simulink model "haya_cvt_multiple_gear"  (R2020a)
settings: Solver=VariableStepAuto  StartTime=0.0  StopTime=10.0  RelTol=1e-3
libraries: fl_lib x19, nesl_utility x9, sdl_lib x9, simulink x2
settings Model: Creator=kishan  LastModifiedBy=kishan

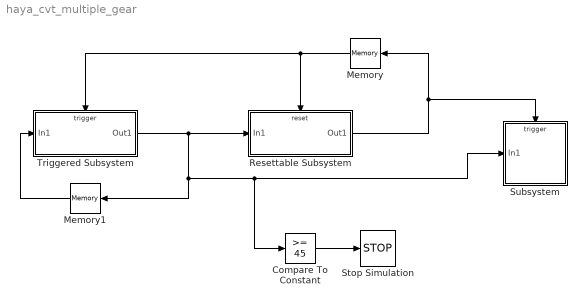
== system haya_cvt_multiple_gear ==
  Compare To Constant : simulink/Logic and Bit Operations/Compare To Constant  relop=>=  const=45  OutDataTypeStr=boolean
  Memory : Memory
  Memory1 : Memory  InitialCondition=6.9
  Resettable Subsystem : Subsystem  TreatAsAtomicUnit=on
  Stop Simulation : Stop
  Subsystem : Subsystem
  Triggered Subsystem : Subsystem  TreatAsAtomicUnit=on
  wires:
  Resettable Subsystem/1(Out1) -> Memory/1, Subsystem/Trigger
  Triggered Subsystem/1(Out1) -> Memory1/1, Compare To Constant/1, Subsystem/1(In1), Resettable Subsystem/1(In1)
  Compare To Constant/1 -> Stop Simulation/1
  Memory/1 -> Triggered Subsystem/Trigger, Resettable Subsystem/Reset
  Memory1/1 -> Triggered Subsystem/1(In1)

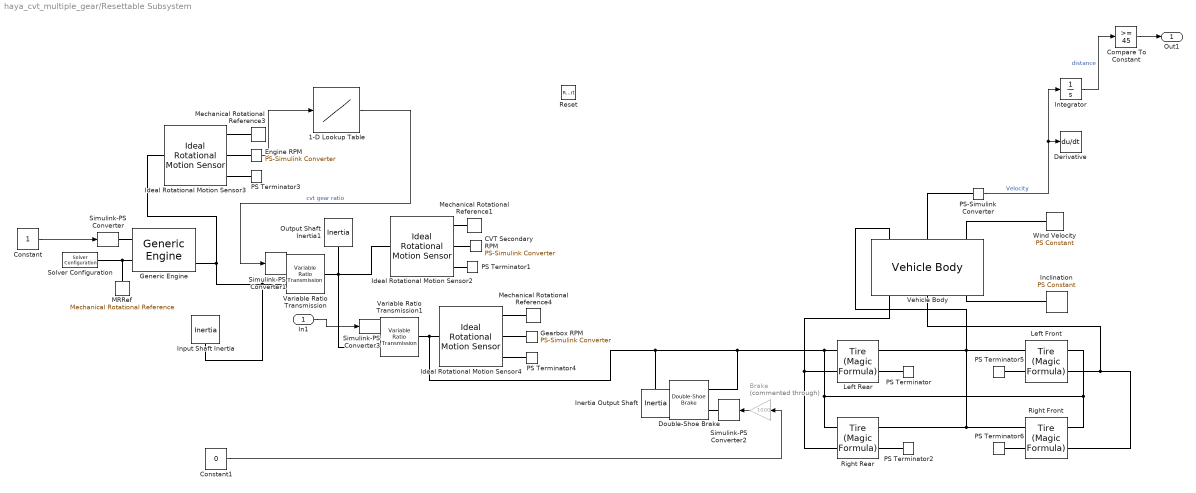
== system haya_cvt_multiple_gear/Resettable Subsystem ==
  In1 : Inport
  Reset : ResetPort  DisableCoverage=on
  1-D Lookup Table : Lookup_n-D  NumberOfTableDimensions=1  BreakpointsForDimension1=[1200, 1300, 1400, 1500, 1600, 1700, 1800, 2000, 2200, 2400, 2600, 2800, 3000, 3200, 3400, 3600, 3800]  Table=[3.9, 3.9, 3.9, 3.9, 3.9, 3.9, 3.9, 3.75, 3.5, 3.2, 2.8, 1.4, 1, 0.9, 0.9, 0.9, 0.9]  InternalRulePriority=Speed  RndMeth=Simplest  InputSameDT=on
  Brake : Gain  Commented=through  Gain=1000
  CVT Secondary RPM : nesl_utility/PS-Simulink Converter  PhysicalDomain=network_engine_domain  SubClassName=ps_output  LeftPortType=input  RightPortType=output  PseudoPeriodic=off  Frequencies=[]  Unit=rpm  AffineConversion=off
  Compare To Constant : simulink/Logic and Bit Operations/Compare To Constant  relop=>=  const=45  OutDataTypeStr=boolean
  Constant : Constant
  Constant1 : Constant  Value=0
  Derivative : Derivative
  Double-Shoe Brake : sdl_lib/Brakes & Detents/Rotational/Double-Shoe Brake  r_drum=150 mm  r_act=100 mm  r_pin=125 mm  theta_pin=15 deg  theta_0=5 deg  theta_shoe=120 deg  mu_visc=.01 N*m/(rad/s)  thermal_port=simscape.enum.thermaleffects.omit  mu=0.3  temperature_TLU=[280.0, 300.0, 320.0] K  mu_TLU=[0.1, 0.05, 0.03]  thermal_mass=50 kJ/K  w_thr=0.01 rad/s  temperature_specify=off  temperature_priority=High  temperature=300 K  temperature_nominal_specify=off  temperature_nominal_unit=K  temperature_nominal_value=1
      settings: SourceProductBaseCode=LD  InternalSimscapePortConfiguration="{\"Bottom\":[],\"Left\":[{\"id\":\"F\",\"label\":\"F\",\"type\":\"input\"},{\"id\":\"S\",\"label\":\"S\",\"type\":\"foundation.mechanical.rotational.rotational\"}],\"Right\":[],\"Top\":[]}"
  Engine RPM : nesl_utility/PS-Simulink Converter  PhysicalDomain=network_engine_domain  SubClassName=ps_output  LeftPortType=input  RightPortType=output  PseudoPeriodic=off  Frequencies=[]  Unit=rpm  AffineConversion=off
  Gearbox RPM : nesl_utility/PS-Simulink Converter  PhysicalDomain=network_engine_domain  SubClassName=ps_output  LeftPortType=input  RightPortType=output  PseudoPeriodic=off  Frequencies=[]  Unit=rpm  AffineConversion=off
  Generic Engine : sdl_lib/Engines/Generic Engine  model_parameterization=2  engine_type=1  P_max=10 HP_DIN  w_P_max=3600 rpm  w_max=3800 rpm  w_min=2000 rpm  w_tab=[1200,1300,1400,1500,1600,1700,1800,1900,1999.91475361355,2037.58825921408,2067.14428302096,2107.1635059702,2136.68404125541,2172.52153339987,2199.90684263059,2233.66234150309,2279.96303278992,2322.09973753281,2353.6667775683,2389.46878119108,2421.01807696573,2463.08380466526,2494.65084470075,2534.65232338915,2583.01726368711,2600,2620.86577206018,2654.46157258512,2711.22546301431,2765.81863886733,2828.84625337326,2893.92037262948,2959.01223614654,3011.45244168423,3074.37359062512,3126.8137961628,3181.31825071162,3235.80496099959,3283.9747144283,3348.94236811948,3390.79516468892,3438.92942959595,3480.79997042623,3535.25119219253,3583.33222431703] rpm  trq_tab=[2.9584703,4.1836314,5.4162917,5.69929300000000,7.851956,9.435718,10.573324,11.506594,12.169014084507,12.7323943661972,13.2394366197183,13.6338028169014,14.0281690140845,14.4788732394366,14.7605633802817,15.2676056338028,15.6056338028169,16.056338028169,16.2816901408451,16.6197183098592,16.7887323943662,17.0140845070423,17.2394366197183,17.5774647887324,17.8028169014085,17.9718309859155,17.9718309859155,18.1971830985916,18.1971830985916,18.5098591549296,19,18.5535211267606,18.2535211267606,18.0845070422535,17.8591549295775,17.6901408450704,17.4084507042254,17.0704225352113,16.6760563380282,16.2816901408451,15.830985915493,15.3239436619718,14.9295774647887,14.4788732394366,13.8028169014085] N*m  pwr_tab=[5.25, 5.75, 6.3, 7, 7.5, 8, 8.4, 8.6, 9] kW  interp_method=simscape.enum.interpolation.smooth  model_inertia=1  inertia=0.8 kg*m^2  initial_velocity=1500 rpm  model_time_constant=1  time_constant=1 s  T0=0  w_thr=100 rpm  idle_speed=1  idle_speed_reference=1500 rpm  tau_controller=1 s  idle_w_thr=1 rpm  redline=1  redline_speed=3550 rpm  tau_redline=1 s  redline_w_thr=1 rpm  fc_model=0  fc_per_rev=25 mg/rev  displaced_volume=400 cm^3  rev_per_cycle=2  fc_w_tab=[1000, 2000, 3000, 4000, 5000, 6000] rpm  fc_trq_tab=[0, 80, 160, 200, 240, 320, 360, 400] N*m  fc_tab=[.5, .9, 1.4, 1.6, 1.9, 2.7, 3.4, 4.4; 1, 1.7, 2.7, 3.1, 3.6, 5, 6, 7.4; 1.4, 2.7, 4, 4.8, 5.6, 7.5, 8.5, 10.5; 2, 3.6, 5.8, 6.7, 8, 10.4, 11.7, 13.3; 2.5, 4.8, 7.9, 9.4, 10.8, 14, 16.2, 18.6; 3.1, 6, 10.3, 11.9, 13.8, 18.4, 22, 26.5] g/s  bmep_tab=[0, 250, 500, 625, 750, 1000, 1150, 1250] kPa  bsfc_tab=[410, 380, 300, 280, 270, 290, 320, 380; 410, 370, 290, 270, 260, 270, 285, 320; 415, 380, 290, 275, 265, 270, 270, 300; 420, 390, 310, 290, 285, 280, 280, 285; 430, 410, 340, 320, 310, 300, 310, 320; 450, 430, 370, 340, 330, 330, 350, 380] g/hr/kW  fc_interp_method=simscape.enum.interpolation.linear
      settings: SourceProductBaseCode=LD  LogSimulationData=on  InternalSimscapePortConfiguration="{\"Bottom\":[],\"Left\":[{\"id\":\"T\",\"label\":\"T\",\"type\":\"input\"},{\"id\":\"B\",\"label\":\"B\",\"type\":\"foundation.mechanical.rotational.rotational\"}],\"Right\":[{\"id\":\"P\",\"label\":\"P\",\"type\":\"output\"},{\"id\":\"FC\",\"label\":\"FC\",\"type\":\"output\"},{\"id\":\"F\",\"label\":\"F\",\"type\":\"foundation.mechanical.rotational.rotational\"}],\"Top\":[]}"
  Ideal Rotational Motion Sensor2 : fl_lib/Mechanical/Mechanical Sensors/Ideal Rotational Motion Sensor  wrap_angle=simscape.enum.onoff.off  offset=0 rad
  Ideal Rotational Motion Sensor3 : fl_lib/Mechanical/Mechanical Sensors/Ideal Rotational Motion Sensor  wrap_angle=simscape.enum.onoff.off  offset=0 rad
  Ideal Rotational Motion Sensor4 : fl_lib/Mechanical/Mechanical Sensors/Ideal Rotational Motion Sensor  wrap_angle=simscape.enum.onoff.off  offset=0 rad
  Inclination : fl_lib/Physical Signals/Sources/PS Constant  constant=0
  Inertia Output Shaft : fl_lib/Mechanical/Rotational Elements/Inertia  inertia=1e-1 kg*m^2  w_specify=on  w_priority=High  w=0 rpm  w_nominal_specify=off  w_nominal_unit=rad/s  w_nominal_value=1  t_specify=off  t_priority=High  t=0 N*m  t_nominal_specify=off  t_nominal_unit=N*m  t_nominal_value=1
  Input Shaft Inertia : fl_lib/Mechanical/Rotational Elements/Inertia  inertia=0.00253 kg*m^2  w_specify=on  w_priority=None  w=2500 rpm  w_nominal_specify=off  w_nominal_unit=rad/s  w_nominal_value=1  t_specify=off  t_priority=High  t=0 N*m  t_nominal_specify=off  t_nominal_unit=N*m  t_nominal_value=1
  Integrator : Integrator
  Left Front : sdl_lib/Tires & Vehicles/Tire (Magic Formula)  parameterization=sdl.enum.magic_tire_model.constant  F_z1=3000 N  F_x1=3500 N  kappa1=10  B_m=5  C_m=2  D_m=0.3  E_m=1  fz0=4000 N  p_Cx=1.685  p_Dx=[1.21, -.037]  p_Ex=[.344, .095, -.02, 0]  p_Kx=[21.51, -.163, .245]  p_Hx=[-.002, .002]  p_Vx=[0, 0]  v_tr_thr=0.1 m/s  r_e=0.292 m  model_compliance=0  stiffness=1e6 N/m  damping=1000 N/(m/s)  model_inertia=1  inertia=0.0667255 kg*m^2  initial_velocity=0 rpm  model_resistance=1  resistance_model=1  coeff=0.02  p_tire=250e3 Pa  alpha=-0.003  beta=0.97  coeff_a=84e-4  coeff_b=6.2e-4 s/m  coeff_c=1.6e-4 s^2/m^2  v_thr=0.001 m/s
  Left Rear : sdl_lib/Tires & Vehicles/Tire (Magic Formula)  parameterization=sdl.enum.magic_tire_model.constant  F_z1=3000 N  F_x1=3500 N  kappa1=10  B_m=5  C_m=2  D_m=0.3  E_m=1  fz0=4000 N  p_Cx=1.685  p_Dx=[1.21, -.037]  p_Ex=[.344, .095, -.02, 0]  p_Kx=[21.51, -.163, .245]  p_Hx=[-.002, .002]  p_Vx=[0, 0]  v_tr_thr=0.1 m/s  r_e=0.292 m  model_compliance=0  stiffness=1e6 N/m  damping=1000 N/(m/s)  model_inertia=1  inertia=0.0667255 kg*m^2  initial_velocity=0 rpm  model_resistance=1  resistance_model=1  coeff=0.02  p_tire=250e3 Pa  alpha=-0.003  beta=0.97  coeff_a=84e-4  coeff_b=6.2e-4 s/m  coeff_c=1.6e-4 s^2/m^2  v_thr=0.001 m/s
  MRRef : fl_lib/Mechanical/Rotational Elements/Mechanical Rotational Reference
  Mechanical Rotational Reference1 : fl_lib/Mechanical/Rotational Elements/Mechanical Rotational Reference
  Mechanical Rotational Reference3 : fl_lib/Mechanical/Rotational Elements/Mechanical Rotational Reference
  Mechanical Rotational Reference4 : fl_lib/Mechanical/Rotational Elements/Mechanical Rotational Reference
  Output Shaft Inertia1 : fl_lib/Mechanical/Rotational Elements/Inertia  inertia=0.00243 kg*m^2  w_specify=on  w_priority=None  w=2500 rpm  w_nominal_specify=off  w_nominal_unit=rad/s  w_nominal_value=1  t_specify=off  t_priority=High  t=0 N*m  t_nominal_specify=off  t_nominal_unit=N*m  t_nominal_value=1
  PS Terminator{,1..6} (7 alike) : fl_lib/Physical Signals/Sinks/PS Terminator
  PS-Simulink Converter : nesl_utility/PS-Simulink Converter  PhysicalDomain=network_engine_domain  SubClassName=ps_output  LeftPortType=input  RightPortType=output  PseudoPeriodic=off  Frequencies=[]  Unit=km/hr  AffineConversion=off
  Right Front : sdl_lib/Tires & Vehicles/Tire (Magic Formula)  parameterization=sdl.enum.magic_tire_model.constant  F_z1=3000 N  F_x1=3500 N  kappa1=10  B_m=5  C_m=2  D_m=0.3  E_m=1  fz0=4000 N  p_Cx=1.685  p_Dx=[1.21, -.037]  p_Ex=[.344, .095, -.02, 0]  p_Kx=[21.51, -.163, .245]  p_Hx=[-.002, .002]  p_Vx=[0, 0]  v_tr_thr=0.1 m/s  r_e=0.292 m  model_compliance=0  stiffness=1e6 N/m  damping=1000 N/(m/s)  model_inertia=1  inertia=0.0667255 kg*m^2  initial_velocity=0 rpm  model_resistance=1  resistance_model=1  coeff=0.02  p_tire=250e3 Pa  alpha=-0.003  beta=0.97  coeff_a=84e-4  coeff_b=6.2e-4 s/m  coeff_c=1.6e-4 s^2/m^2  v_thr=0.001 m/s
  Right Rear : sdl_lib/Tires & Vehicles/Tire (Magic Formula)  parameterization=sdl.enum.magic_tire_model.constant  F_z1=3000 N  F_x1=3500 N  kappa1=10  B_m=5  C_m=2  D_m=0.3  E_m=1  fz0=4000 N  p_Cx=1.685  p_Dx=[1.21, -.037]  p_Ex=[.344, .095, -.02, 0]  p_Kx=[21.51, -.163, .245]  p_Hx=[-.002, .002]  p_Vx=[0, 0]  v_tr_thr=0.1 m/s  r_e=0.292 m  model_compliance=0  stiffness=1e6 N/m  damping=1000 N/(m/s)  model_inertia=1  inertia=0.0667255 kg*m^2  initial_velocity=0 rpm  model_resistance=1  resistance_model=1  coeff=0.02  p_tire=250e3 Pa  alpha=-0.003  beta=0.97  coeff_a=84e-4  coeff_b=6.2e-4 s/m  coeff_c=1.6e-4 s^2/m^2  v_thr=0.001 m/s
  Simulink-PS Converter : nesl_utility/Simulink-PS Converter  PhysicalDomain=network_engine_domain  SubClassName=ps_input  LeftPortType=input  RightPortType=output  PseudoPeriodic=off  Frequencies=[]  NoiseDistribution=none  NoiseParameters=[]  Unit=1  AffineConversion=off  FilteringAndDerivatives=zero  SimscapeFilterOrder=1  InputFilterTimeConstant=0.001  UdotUserProvided=1
  Simulink-PS Converter1 : nesl_utility/Simulink-PS Converter  PhysicalDomain=network_engine_domain  SubClassName=ps_input  LeftPortType=input  RightPortType=output  PseudoPeriodic=off  Frequencies=[]  NoiseDistribution=none  NoiseParameters=[]  Unit=1  AffineConversion=off  FilteringAndDerivatives=zero  SimscapeFilterOrder=1  InputFilterTimeConstant=.001  UdotUserProvided=0
  Simulink-PS Converter2 : nesl_utility/Simulink-PS Converter  PhysicalDomain=network_engine_domain  SubClassName=ps_input  LeftPortType=input  RightPortType=output  PseudoPeriodic=off  Frequencies=[]  NoiseDistribution=none  NoiseParameters=[]  Unit=N  AffineConversion=off  FilteringAndDerivatives=zero  SimscapeFilterOrder=1  InputFilterTimeConstant=0.001  UdotUserProvided=1
  Simulink-PS Converter3 : nesl_utility/Simulink-PS Converter  PhysicalDomain=network_engine_domain  SubClassName=ps_input  LeftPortType=input  RightPortType=output  PseudoPeriodic=off  Frequencies=[]  NoiseDistribution=none  NoiseParameters=[]  Unit=1  AffineConversion=off  FilteringAndDerivatives=zero  SimscapeFilterOrder=1  InputFilterTimeConstant=0.001  UdotUserProvided=1
  Solver Configuration : nesl_utility/Solver Configuration  PhysicalDomain=network_engine_domain  SubClassName=solver  LeftPortType=input  RightPortType=generic  Tones=[]  Harmonics=[]  SimulateNoise=off  Profile=off  UseLocalSampling=off  EnableSwitchedLinearOptims=on  FrequencyDomain=off  UseCCode=off  RelTol=0.001  AbsTol=1e-06  MinStep=1e-09  ToWorkspace=off  RevertToSquareIcSolve=off  NumHomotopyIterations=100  PhasorMode=off  PhasorModeNumHarmonics=1  DoDC=off  ResidualTolerance=1e-9  UseLocalSolver=off  LocalSolverChoice=NE_BACKWARD_EULER_ADVANCER  LocalSolverSampleTime=0.001  DoFixedCost=off  MaxNonlinIter=3  MaxModeIter=2  LinearAlgebra=Sparse  EquationFormulation=NE_TIME_EF  DelaysMemoryBudget=1024  AutomaticFiltering=on  FilteringTimeConstant=0.001  PartitionStorageMethod=AS_NEEDED  PartitionMemoryBudget=1024  PartitionMethod=FAST
  Variable Ratio Transmission : sdl_lib/Couplings & Drives/Variable Ratio Transmission  rotation_direction=1  kp=3e5 N*m/rad  kv=0.05 N*m/(rad/s)  initial_torque=0 N*m  losses_model=2  efficiency=0.8  mu_visc=[0, 0] N*m/(rad/s)  w_thr=0.01 rad/s  R_specify=off  R_priority=None  R=1  R_nominal_specify=off  R_nominal_unit=1  R_nominal_value=1
      settings: SourceProductBaseCode=LD  InternalSimscapePortConfiguration="{\"Bottom\":[],\"Left\":[{\"id\":\"ratio\",\"label\":\"r\",\"type\":\"input\"},{\"id\":\"B\",\"label\":\"B\",\"type\":\"foundation.mechanical.rotational.rotational\"}],\"Right\":[{\"id\":\"F\",\"label\":\"F\",\"type\":\"foundation.mechanical.rotational.rotational\"}],\"Top\":[]}"
  Variable Ratio Transmission1 : sdl_lib/Couplings & Drives/Variable Ratio Transmission  rotation_direction=1  kp=3e5 N*m/rad  kv=0.05 N*m/(rad/s)  initial_torque=0 N*m  losses_model=2  efficiency=0.8  mu_visc=[0, 0] N*m/(rad/s)  w_thr=0.01 rad/s  R_specify=off  R_priority=None  R=1  R_nominal_specify=off  R_nominal_unit=1  R_nominal_value=1
      settings: SourceProductBaseCode=LD  InternalSimscapePortConfiguration="{\"Bottom\":[],\"Left\":[{\"id\":\"ratio\",\"label\":\"r\",\"type\":\"input\"},{\"id\":\"B\",\"label\":\"B\",\"type\":\"foundation.mechanical.rotational.rotational\"}],\"Right\":[{\"id\":\"F\",\"label\":\"F\",\"type\":\"foundation.mechanical.rotational.rotational\"}],\"Top\":[]}"
  Vehicle Body : sdl_lib/Tires & Vehicles/Vehicle Body  mass=250 kg  n_w=2  x_f=770.98 mm  x_r=639.02 mm  y_c=491.9 mm  mass_var=simscape.enum.onoff.off  model_pitch=simscape.enum.onoff.off  inertia=4000 kg*m^2  suspension_model=sdl.enum.linearTLU.linear  k_f=1e4 N/m  b_f=1e4 N/(m/s)  k_r=1e4 N/m  b_r=1e4 N/(m/s)  k_f_TLU=[-2000, -1000, 0, 1000, 2000] N  x_f_TLU=[-.4, -.2, 0, .2, .4] m  b_f_TLU=[-200, -100, 0, 100, 200] N  v_f_TLU=[-4, -2, 0, 2, 4] m/s  k_r_TLU=[-2000, -1000, 0, 1000, 2000] N  x_r_TLU=[-.4, -.2, 0, .2, .4] m  b_r_TLU=[-200, -100, 0, 100, 200] N  v_r_TLU=[-4, -2, 0, 2, 4] m/s  interp_method=simscape.enum.interpolation.linear  extrap_method=simscape.enum.extrapolation.linear  model_hardstop=simscape.enum.onoff.off  upper_bound_f=.25 m  lower_bound_f=-.25 m  stop_k_f=1e6 N/m  stop_b_f=150 N/(m/s)  upper_bound_r=.25 m  lower_bound_r=-.25 m  stop_k_r=1e6 N/m  stop_b_r=150 N/(m/s)  initial_pitch=0 rad  initial_pitch_rate=0 rad/s  g=9.81 m/s^2  liftoff_warning=simscape.enum.onoff.off  area=0.8 m^2  Cd=1.2  rho=1.18 kg/m^3  v_specify=off  v_priority=High  v=0 m/s  v_nominal_specify=off  v_nominal_unit=m/s  v_nominal_value=1
      settings: LogSimulationData=on
  Wind Velocity : fl_lib/Physical Signals/Sources/PS Constant  constant=0
  Out1 : Outport
  wires:
  PS-Simulink Converter/1 -> Derivative/1, Integrator/1  "Velocity"
  1-D Lookup Table/1 -> Simulink-PS Converter1/1  "cvt gear ratio"
  Brake/1 -> Simulink-PS Converter2/1
  Compare To Constant/1 -> Out1/1
  Engine RPM/1 -> 1-D Lookup Table/1
  Constant/1 -> Simulink-PS Converter/1
  Constant1/1 -> Brake/1
  Integrator/1 -> Compare To Constant/1  "distance"
  In1/1 -> Simulink-PS Converter3/1
  connections:
  Right Rear/RConn2 -- Right Front/RConn2 -- Left Front/RConn2 -- Left Rear/RConn2 -- Vehicle Body/LConn1
  Right Front/LConn1 -- Vehicle Body/RConn2 -- Left Front/LConn1
  Double-Shoe Brake/LConn2 -- Variable Ratio Transmission1/RConn1 -- Ideal Rotational Motion Sensor4/LConn1 -- Inertia Output Shaft/LConn1 -- Left Rear/LConn2 -- Right Front/LConn2 -- Left Front/LConn2 -- Right Rear/LConn2
  Ideal Rotational Motion Sensor2/LConn1 -- Variable Ratio Transmission1/LConn2 -- Variable Ratio Transmission/RConn1 -- Output Shaft Inertia1/LConn1
  Variable Ratio Transmission/LConn2 -- Input Shaft Inertia/LConn1 -- Generic Engine/RConn3 -- Ideal Rotational Motion Sensor3/LConn1
  Right Rear/LConn1 -- Vehicle Body/RConn1 -- Left Rear/LConn1
  MRRef/LConn1 -- Generic Engine/LConn2 -- Solver Configuration/RConn1
  PS Terminator/LConn1 -- Left Rear/RConn1
  PS Terminator5/LConn1 -- Left Front/RConn1
  Gearbox RPM/LConn1 -- Ideal Rotational Motion Sensor4/RConn2
  Mechanical Rotational Reference3/LConn1 -- Ideal Rotational Motion Sensor3/RConn1
  Simulink-PS Converter1/RConn1 -- Variable Ratio Transmission/LConn1
  PS-Simulink Converter/LConn1 -- Vehicle Body/LConn2
  PS Terminator1/LConn1 -- Ideal Rotational Motion Sensor2/RConn3
  Inclination/RConn1 -- Vehicle Body/RConn3
  Wind Velocity/RConn1 -- Vehicle Body/LConn3
  Double-Shoe Brake/LConn1 -- Simulink-PS Converter2/RConn1
  Mechanical Rotational Reference4/LConn1 -- Ideal Rotational Motion Sensor4/RConn1
  CVT Secondary RPM/LConn1 -- Ideal Rotational Motion Sensor2/RConn2
  Simulink-PS Converter/RConn1 -- Generic Engine/LConn1
  PS Terminator2/LConn1 -- Right Rear/RConn1
  PS Terminator4/LConn1 -- Ideal Rotational Motion Sensor4/RConn3
  PS Terminator6/LConn1 -- Right Front/RConn1
  Mechanical Rotational Reference1/LConn1 -- Ideal Rotational Motion Sensor2/RConn1
  Engine RPM/LConn1 -- Ideal Rotational Motion Sensor3/RConn2
  PS Terminator3/LConn1 -- Ideal Rotational Motion Sensor3/RConn3
  Simulink-PS Converter3/RConn1 -- Variable Ratio Transmission1/LConn1

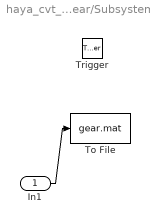
== system haya_cvt_multiple_gear/Subsystem ==
  In1 : Inport
  Trigger : TriggerPort  VariantControl=Variant  PortDimensions=1
  To File : ToFile  Filename=gear.mat  SaveFormat=Timeseries
  wires:
  In1/1 -> To File/1

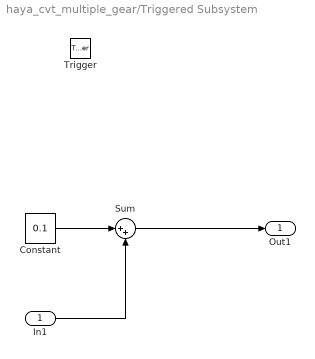
== system haya_cvt_multiple_gear/Triggered Subsystem ==
  In1 : Inport
  Trigger : TriggerPort  VariantControl=Variant
  Constant : Constant  Value=0.1
  Sum : Sum  Inputs=|++
  Out1 : Outport
  wires:
  Constant/1 -> Sum/1
  Sum/1 -> Out1/1
  In1/1 -> Sum/2
